simulink model "CardioPumpModel"  (R2019b)
settings: Solver=VariableStepAuto  StartTime=0.0  StopTime=10.0  RelTol=1e-3
settings Model: Creator=SÜLEYMAN  LastModifiedBy=SÜLEYMAN

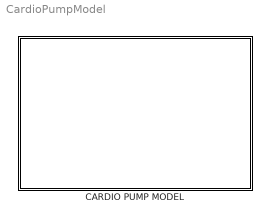
== system CardioPumpModel ==
  CARDIO PUMP MODEL : Subsystem

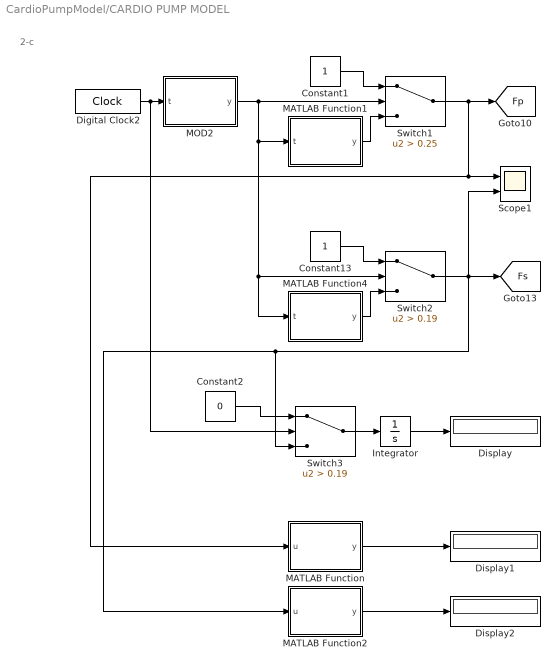
== system CardioPumpModel/CARDIO PUMP MODEL ==
  note: 2-c
  Constant1 : Constant
  Constant13 : Constant
  Constant2 : Constant  Value=0
  Digital Clock2 : DigitalClock  SampleTime=0.001
  Display : Display
  Display1 : Display
  Display2 : Display
  Integrator : Integrator
  MATLAB Function : MATLAB Function  TreatAsAtomicUnit=on
  MATLAB Function1 : MATLAB Function  TreatAsAtomicUnit=on
  MATLAB Function2 : MATLAB Function  TreatAsAtomicUnit=on
  MATLAB Function4 : MATLAB Function  TreatAsAtomicUnit=on
  MOD2 : MATLAB Function  TreatAsAtomicUnit=on
  Scope1 : Scope  NumInputPorts=2
  Switch1 : Switch  Criteria=u2 > Threshold  Threshold=0.25
  Switch2 : Switch  Criteria=u2 > Threshold  Threshold=0.19
  Switch3 : Switch  Criteria=u2 > Threshold  Threshold=0.19
  tag scope: Fp=global, Fs=global
  wires:
  Constant13/1 -> Switch2/1
  MOD2/1(y) -> MATLAB Function4/1(t), Switch2/2, MATLAB Function1/1(t), Switch1/2
  Switch1/1 -> [Fp], MATLAB Function/1(u), Scope1/1
  Switch2/1 -> MATLAB Function2/1(u), Switch3/3, Scope1/2, [Fs]
  Digital Clock2/1 -> Switch3/2, MOD2/1(t)
  MATLAB Function4/1(y) -> Switch2/3
  Constant1/1 -> Switch1/1
  MATLAB Function1/1(y) -> Switch1/3
  Constant2/1 -> Switch3/1
  Switch3/1 -> Integrator/1
  Integrator/1 -> Display/1
  MATLAB Function2/1(y) -> Display2/1
  MATLAB Function/1(y) -> Display1/1

== matlab function CardioPumpModel/CARDIO PUMP MODEL/MATLAB Function1 ==
  data: t input; y output
function y = fcn(t)
y = (abs((sin(pi*t/0.25)))^1.55)*460+1;

== matlab function CardioPumpModel/CARDIO PUMP MODEL/MATLAB Function4 ==
  data: t input; y output
function y = fcn(t)
y = (abs((sin(pi*t/0.19)))^2)*670+1;

== matlab function CardioPumpModel/CARDIO PUMP MODEL/MOD2 ==
  data: t input; y output
function y = fcn(t)
    period=mod(t,0.84);
y = period;

== matlab function CardioPumpModel/CARDIO PUMP MODEL/MATLAB Function ==
  data: u input; y output
function y = fcn(u)

y = abs(fft(u,length(u)));

== matlab function CardioPumpModel/CARDIO PUMP MODEL/MATLAB Function2 ==
  data: u input; y output
function y = fcn(u)

y = abs(fft(u,length(u)));
